simulink model "BloodPressure_ADC1"  (R2020b)
settings: Solver=ode15s  StartTime=0.0  StopTime=55  RelTol=1e-3  AbsTol=1e-3  EnableMultiTasking=on
libraries: fl_lib x33, nesl_utility x7, ee_lib x7
CloseFcn:
  | try,close(h1_elec_strain_gauge),end
  | clear h1_elec_strain_gauge
  | 
  | clear logsout_elec_strain_gauge
  | clear simlog_elec_strain_gauge
  | clear tout
Description:
  | Strain Gauge and Wheatstone Bridge
  | 
  | Copyright 2008-2018 The MathWorks, Inc.
settings Model: ExtModeAutoUpdateStatusClock=off  Creator=MathWorks  LastModifiedBy=bolic
settings SolverCC: AutoScaleAbsTol=off
settings DataIOCC: MaxDataPoints=10000  ReturnWorkspaceOutputs=off  SignalLoggingName=logsout_elec_strain_gauge  Refine=5
settings OptimizationCC: ExpressionDepthLimit=2147483647  InitFltsAndDblsToZero=on  LifeSpan=inf
settings DebuggingCC: SaveWithParameterizedLinksMsg=none  UnderspecifiedInitializationDetection=Classic  MergeDetectMultiDrivingBlocksExec=none  SignalResolutionControl=TryResolveAllWithWarning  FcnCallInpInsideContextMsg=warning  StateNameClashWarn=warning  SFUnexpectedBacktrackingDiag=warning  SFNoUnconditionalDefaultTransitionDiag=warning  SFExecutionAtInitializationDiag=none  ArithmeticOperatorsInVariantConditions=warning
settings HardwareCC: ProdBitPerPointer=32  ProdBitPerSizeT=32  ProdBitPerPtrDiffT=32  ProdLargestAtomicFloat=None  ProdIntDivRoundTo=Undefined  ProdEndianess=Unspecified  ProdWordSize=32  ProdHWDeviceType=32-bit Generic
settings ModelReferenceCC: PropagateSignalLabelsOutOfModel=off
settings SFSimCC: SimUseLocalCustomCode=off  CustomCodeUndefinedFunction=UseInterfaceOnly
settings RTWCC: RTWUseLocalCustomCode=off
settings CodeAppCC: StateflowObjectComments=on
settings GRTTargetCC: TargetFcnLib=ansi_tfl_tmw.mat  TargetLangStandard=C89/C90 (ANSI)  CombineOutputUpdateFcns=off  GRTInterface=on
settings ConfigComp: CovMetricSettings=dw  CovSaveCumulativeToWorkspaceVar=on  CovSaveSingleToWorkspaceVar=on  CovExternalEMLEnable=off  CovSFcnEnable=off
settings SimscapeCC: SimscapeLogType=all  SimscapeLogSimulationStatistics=on  SimscapeLogName=simlog_elec_strain_gauge  SimscapeLogDataHistory=10000

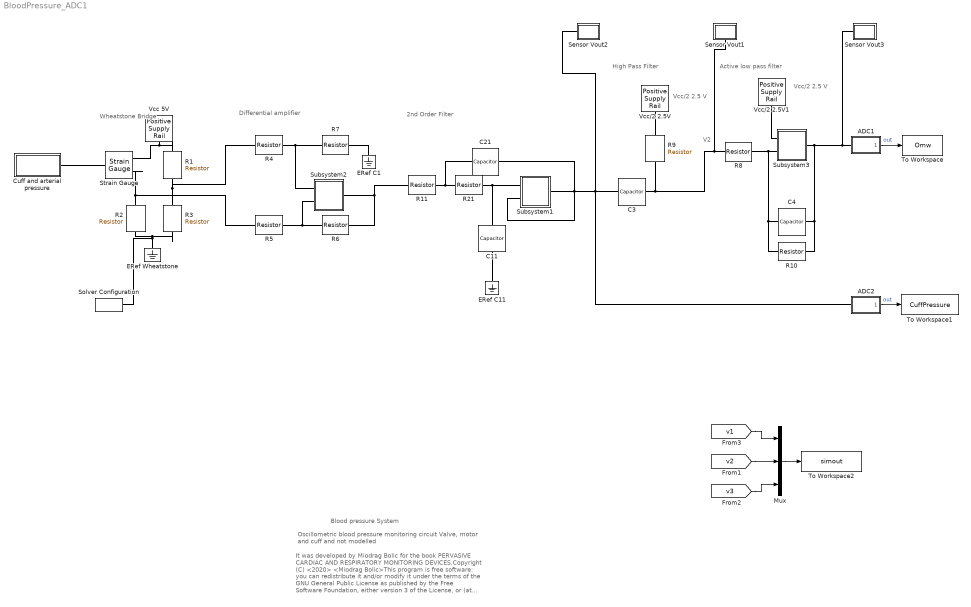
== system BloodPressure_ADC1 ==
  note: Vcc/2
      | 2.5 V
  note: It was developed by Miodrag Bolic for the book PERVASIVE CARDIAC AND RESPIRATORY MONITORING DEVICES.Copyright (C) <2020> <Miodrag Bolic>This program is free software: you can redistribute it and/or modify it under the terms of the GNU General Public License as published by the Free Software Foundation, either version 3 of the License, or (at your option) any later version. This program is distributed in the hope that it will be useful, but WITHOUT ANY WARRANTY; without even the implied warranty of MERCHANTABILITY or FITNESS FOR A PARTICULAR PURPOSE. See the GNU General Public License for more details <https://www.gnu.org/licenses/>.
  note: Wheatstone
      | Bridge
  note: Oscillometric blood pressure monitoring circuit
      | Valve, motor and cuff and not modelled
  note: 2nd Order Filter
  note: V2
  note: High Pass Filter
  note: Active low pass filter
  note: Blood pressure System
  note: Differential amplifier
  note: Vcc/2
      | 2.5 V
  ADC1 : Subsystem  mask(ADC){fs=200, N=12, vmax=5, ileak=1e-9, C=10e-12}
      mask prompts: fs "Sampling rate (Hz)"; N "Number of bits"; vmax "Input voltage for max output (V)"; ileak "Leakage current (A)"; C "Pin capacitance (F)"
      mask help: Simplified analog-to-digital converter
  ADC2 : Subsystem  mask(ADC){fs=200, N=12, vmax=5, ileak=1e-9, C=10e-12}
      mask prompts: fs "Sampling rate (Hz)"; N "Number of bits"; vmax "Input voltage for max output (V)"; ileak "Leakage current (A)"; C "Pin capacitance (F)"
      mask help: Simplified analog-to-digital converter
  C11 : fl_lib/Electrical/Electrical Elements/Capacitor  c=800 nF  r=0 Ohm  g=0 1/Ohm  i_specify=off  i_priority=High  i=0 A  i_nominal_specify=off  i_nominal_unit=A  i_nominal_value=1  v_specify=off  v_priority=High  v=0 V  v_nominal_specify=off  v_nominal_unit=V  v_nominal_value=1  vc_specify=off  vc_priority=High  vc=0 V  vc_nominal_specify=off  vc_nominal_unit=V  vc_nominal_value=1
      settings: AttributesFormatString=%<c> %<c_unit>  SourceProductName=Foundation Library
  C21 : fl_lib/Electrical/Electrical Elements/Capacitor  c=800 nF  r=0 Ohm  g=0 1/Ohm  i_specify=off  i_priority=High  i=0 A  i_nominal_specify=off  i_nominal_unit=A  i_nominal_value=1  v_specify=off  v_priority=High  v=0 V  v_nominal_specify=off  v_nominal_unit=V  v_nominal_value=1  vc_specify=off  vc_priority=High  vc=0 V  vc_nominal_specify=off  vc_nominal_unit=V  vc_nominal_value=1
      settings: AttributesFormatString=%<c>%<c_unit>  SourceProductName=Foundation Library
  C3 : fl_lib/Electrical/Electrical Elements/Capacitor  c=3.3 uF  r=1e-6 Ohm  g=0 1/Ohm  i_specify=off  i_priority=None  i=0 A  i_nominal_specify=off  i_nominal_unit=A  i_nominal_value=1  v_specify=off  v_priority=None  v=0 V  v_nominal_specify=off  v_nominal_unit=V  v_nominal_value=1  vc_specify=off  vc_priority=High  vc=0 V  vc_nominal_specify=off  vc_nominal_unit=V  vc_nominal_value=1
      settings: AttributesFormatString=%<c>%<c_unit>
  C4 : fl_lib/Electrical/Electrical Elements/Capacitor  c=0.6 nF  r=1e-6 Ohm  g=0 1/Ohm  i_specify=off  i_priority=None  i=0 A  i_nominal_specify=off  i_nominal_unit=A  i_nominal_value=1  v_specify=off  v_priority=None  v=0 V  v_nominal_specify=off  v_nominal_unit=V  v_nominal_value=1  vc_specify=off  vc_priority=High  vc=0 V  vc_nominal_specify=off  vc_nominal_unit=V  vc_nominal_value=1
      settings: AttributesFormatString=%<c>%<c_unit>
  Cuff and arterial pressure : Subsystem
  ERef C1 : fl_lib/Electrical/Electrical Elements/Electrical Reference
      settings: SourceProductName=Foundation Library
  ERef C11 : fl_lib/Electrical/Electrical Elements/Electrical Reference
      settings: SourceProductName=Foundation Library
  ERef Wheatstone : fl_lib/Electrical/Electrical Elements/Electrical Reference
      settings: SourceProductName=Foundation Library
  Mux : Mux  Inputs=3
  R1 : fl_lib/Electrical/Electrical Elements/Resistor  R=120 Ohm  i_specify=off  i_priority=High  i=0 A  i_nominal_specify=off  i_nominal_unit=A  i_nominal_value=1  v_specify=off  v_priority=High  v=0 V  v_nominal_specify=off  v_nominal_unit=V  v_nominal_value=1
      settings: AttributesFormatString=%<R> %<R_unit>  SourceProductName=Foundation Library
  R10 : fl_lib/Electrical/Electrical Elements/Resistor  R=15 MOhm  i_specify=off  i_priority=None  i=0 A  i_nominal_specify=off  i_nominal_unit=A  i_nominal_value=1  v_specify=off  v_priority=None  v=0 V  v_nominal_specify=off  v_nominal_unit=V  v_nominal_value=1
      settings: AttributesFormatString=%<R>%<R_unit>
  R11 : fl_lib/Electrical/Electrical Elements/Resistor  R=10 kOhm  i_specify=off  i_priority=High  i=0 A  i_nominal_specify=off  i_nominal_unit=A  i_nominal_value=1  v_specify=off  v_priority=High  v=0 V  v_nominal_specify=off  v_nominal_unit=V  v_nominal_value=1
      settings: AttributesFormatString=%<R> %<R_unit>  SourceProductName=Foundation Library
  R2 : fl_lib/Electrical/Electrical Elements/Resistor  R=120 Ohm  i_specify=off  i_priority=High  i=0 A  i_nominal_specify=off  i_nominal_unit=A  i_nominal_value=1  v_specify=off  v_priority=High  v=0 V  v_nominal_specify=off  v_nominal_unit=V  v_nominal_value=1
      settings: AttributesFormatString=%<R> %<R_unit>  SourceProductName=Foundation Library
  R21 : fl_lib/Electrical/Electrical Elements/Resistor  R="10  kOhm"  i_specify=off  i_priority=High  i=0 A  i_nominal_specify=off  i_nominal_unit=A  i_nominal_value=1  v_specify=off  v_priority=High  v=0 V  v_nominal_specify=off  v_nominal_unit=V  v_nominal_value=1
      settings: AttributesFormatString=%<R>%<R_unit>  SourceProductName=Foundation Library
  R3 : fl_lib/Electrical/Electrical Elements/Resistor  R=120 Ohm  i_specify=off  i_priority=High  i=0 A  i_nominal_specify=off  i_nominal_unit=A  i_nominal_value=1  v_specify=off  v_priority=High  v=0 V  v_nominal_specify=off  v_nominal_unit=V  v_nominal_value=1
      settings: AttributesFormatString=%<R> %<R_unit>  SourceProductName=Foundation Library
  R4 : fl_lib/Electrical/Electrical Elements/Resistor  R=100 Ohm  i_specify=off  i_priority=None  i=0 A  i_nominal_specify=off  i_nominal_unit=A  i_nominal_value=1  v_specify=off  v_priority=None  v=0 V  v_nominal_specify=off  v_nominal_unit=V  v_nominal_value=1
      settings: AttributesFormatString=%<R> %<R_unit>
  R5 : fl_lib/Electrical/Electrical Elements/Resistor  R=100 Ohm  i_specify=off  i_priority=None  i=0 A  i_nominal_specify=off  i_nominal_unit=A  i_nominal_value=1  v_specify=off  v_priority=None  v=0 V  v_nominal_specify=off  v_nominal_unit=V  v_nominal_value=1
      settings: AttributesFormatString=%<R> %<R_unit>
  R6 : fl_lib/Electrical/Electrical Elements/Resistor  R=10 kOhm  i_specify=off  i_priority=None  i=0 A  i_nominal_specify=off  i_nominal_unit=A  i_nominal_value=1  v_specify=off  v_priority=None  v=0 V  v_nominal_specify=off  v_nominal_unit=V  v_nominal_value=1
      settings: AttributesFormatString=%<R> %<R_unit>
  R7 : fl_lib/Electrical/Electrical Elements/Resistor  R=10 kOhm  i_specify=off  i_priority=None  i=0 A  i_nominal_specify=off  i_nominal_unit=A  i_nominal_value=1  v_specify=off  v_priority=None  v=0 V  v_nominal_specify=off  v_nominal_unit=V  v_nominal_value=1
      settings: AttributesFormatString=%<R> %<R_unit>
  R8 : fl_lib/Electrical/Electrical Elements/Resistor  R=250 kOhm  i_specify=off  i_priority=None  i=0 A  i_nominal_specify=off  i_nominal_unit=A  i_nominal_value=1  v_specify=off  v_priority=None  v=0 V  v_nominal_specify=off  v_nominal_unit=V  v_nominal_value=1
      settings: AttributesFormatString=%<R>%<R_unit>
  R9 : fl_lib/Electrical/Electrical Elements/Resistor  R=280 kOhm  i_specify=off  i_priority=None  i=0 A  i_nominal_specify=off  i_nominal_unit=A  i_nominal_value=1  v_specify=off  v_priority=None  v=0 V  v_nominal_specify=off  v_nominal_unit=V  v_nominal_value=1
      settings: AttributesFormatString=%<R>%<R_unit>
  Sensor Vout1 : Subsystem
      settings: PortSchema="{\"entries\":[{\"content\":{\"sides\":[{\"content\":{\"connectorIds\":[]},\"type\":\"ConnectorPlacement.EquallySpacedRectSide\",\"uuid\":\"78d8266e-4de3-447e-bfef-e5103e8c82e7\"},{\"content\":{\"connectorIds\":[],\"side\":\"RIGHT\"},\"type\":\"ConnectorPlacement.EquallySpacedRectSide\",\"uuid\":\"24c184c0-4d09-4cde-a27e-d86b719c7490\"},{\"content\":{\"connectorIds\":[],\"side\":\"TOP\"},\"type\":\"ConnectorPlacement.EquallySpacedRectSide\",\"uuid\":\"0a0b328c-c1d1-4c74-810b-0901e018f872\"},{\"content\":{\"connectorIds\":[\"RConn1\"],\"side\":\"BOTTOM\"},\"type\":\"ConnectorPlacement.EquallySpacedRectSide\",\"uuid\":\"04397490-2efd-4059-a127-c3271fe693a1\"},{\"content\":{\"connectorIds\":[],\"side\":\"HIDDEN\"},\"type\":\"ConnectorPlacement.EquallySpacedRectSide\",\"uuid\":\"df448a23-5d4a-4198-9543-ada33aea1d81\"}]},\"type\":\"ConnectorPlacement.EquallySpacedConnector\",\"uuid\":\"43700f0f-07d4-49b8-8a91-5fd2f7a62cdb\"}],\"packageUris\":[\"http://schema.mathworks.com/mf0/Connector/R2020b\"],\"version\":\"1.0\"}"
      mask Display: disp('V')
  Sensor Vout2 : Subsystem
      mask Display: disp('V')
  Sensor Vout3 : Subsystem
      mask Display: disp('V')
  Solver Configuration : nesl_utility/Solver Configuration  PhysicalDomain=network_engine_domain  SubClassName=solver  LeftPortType=input  RightPortType=generic  Tones=[]  Harmonics=[]  SimulateNoise=off  Profile=off  UseLocalSampling=off  EnableSwitchedLinearOptims=on  FrequencyDomain=off  UseCCode=off  RelTol=0.001  AbsTol=1e-06  MinStep=1e-09  ToWorkspace=off  RevertToSquareIcSolve=off  NumHomotopyIterations=100  PhasorMode=off  PhasorModeNumHarmonics=1  DoDC=off  ResidualTolerance=1e-9  UseLocalSolver=off  LocalSolverChoice=NE_BACKWARD_EULER_ADVANCER  LocalSolverSampleTime=.001  DoFixedCost=off  MaxNonlinIter=3  MaxModeIter=2  ComputeImpulses=off  ImpulseIterations=2  LinearAlgebra=auto  EquationFormulation=NE_TIME_EF  DelaysMemoryBudget=1024  AutomaticFiltering=on  FilteringTimeConstant=0.001  PartitionStorageMethod=AS_NEEDED  PartitionMemoryBudget=1024  PartitionMethod=FAST
  Strain Gauge : ee_lib/Sensors & Transducers/Strain Gauge  R=120 Ohm  K=2
      settings: SourceProductBaseCode=PS  InternalSimscapePortConfiguration="{\"Bottom\":[],\"Left\":[{\"id\":\"E\",\"label\":\"E\",\"type\":\"input\"}],\"Right\":[{\"id\":\"p\",\"label\":\"+\",\"type\":\"foundation.electrical.electrical\"},{\"id\":\"n\",\"label\":\"-\",\"type\":\"foundation.electrical.electrical\"}],\"Top\":[]}"
  Subsystem1 : Subsystem
      mask Display: image('op_amp_plus_up.png')
  Subsystem2 : Subsystem
      mask Display: image('op_amp_plus_up.png')
  Subsystem3 : Subsystem
      mask Display: image('op_amp_plus_up.png')
  To Workspace : ToWorkspace  VariableName=Omw  SaveFormat=Timeseries  SampleTime=0.001
  To Workspace1 : ToWorkspace  VariableName=CuffPressure  SaveFormat=Timeseries  SampleTime=0.001
  To Workspace2 : ToWorkspace  VariableName=simout  SaveFormat=Timeseries  SampleTime=-1
  Vcc 5V : ee_lib/Sources/Positive Supply Rail  v0=5 V
      settings: SourceProductBaseCode=PS  InternalSimscapePortConfiguration="{\"Bottom\":[],\"Left\":[],\"Right\":[{\"id\":\"p\",\"label\":\"\",\"type\":\"foundation.electrical.electrical\"}],\"Top\":[]}"
  Vcc/2 2.5V : ee_lib/Sources/Positive Supply Rail  v0=2.5 V
      settings: SourceProductBaseCode=PS  InternalSimscapePortConfiguration="{\"Bottom\":[],\"Left\":[],\"Right\":[{\"id\":\"p\",\"label\":\"\",\"type\":\"foundation.electrical.electrical\"}],\"Top\":[]}"
  Vcc/2 2.5V1 : ee_lib/Sources/Positive Supply Rail  v0=2.5 V
      settings: SourceProductBaseCode=PS  InternalSimscapePortConfiguration="{\"Bottom\":[],\"Left\":[],\"Right\":[{\"id\":\"p\",\"label\":\"\",\"type\":\"foundation.electrical.electrical\"}],\"Top\":[]}"
  wires:
  ADC1/1(Out_Int) -> To Workspace/1  "out"
  ADC2/1(Out_Int) -> To Workspace1/1  "out"
  Mux/1 -> To Workspace2/1
  [v1] -> Mux/1
  [v2] -> Mux/2
  [v3] -> Mux/3
  connections:
  R1/LConn1 -- Strain Gauge/RConn1 -- Vcc 5V/RConn1
  R3/RConn1 -- R2/RConn1 -- Solver Configuration/RConn1 -- ERef Wheatstone/LConn1
  R21/RConn1 -- Subsystem1/LConn1 -- C11/LConn1
  R21/LConn1 -- R11/RConn1 -- C21/LConn1
  C21/RConn1 -- Subsystem1/LConn2 -- Subsystem1/RConn1 -- Sensor Vout2/LConn1 -- C3/LConn1 -- ADC2/LConn1
  R10/RConn1 -- Subsystem3/RConn1 -- Sensor Vout3/LConn1 -- ADC1/LConn1 -- C4/LConn1
  C3/RConn1 -- R9/RConn1 -- Sensor Vout1/RConn1 -- R8/LConn1
  R8/RConn1 -- Subsystem3/LConn2 -- R10/LConn1 -- C4/RConn1
  Vcc/2 2.5V1/RConn1 -- Subsystem3/LConn1
  Vcc/2 2.5V/RConn1 -- R9/LConn1
  Cuff and arterial pressure/RConn1 -- Strain Gauge/LConn1
  ERef C1/LConn1 -- R7/RConn1
  R5/RConn1 -- Subsystem2/LConn2 -- R6/LConn1
  R11/LConn1 -- Subsystem2/RConn1 -- R6/RConn1
  R1/RConn1 -- R4/LConn1 -- R3/LConn1
  R4/RConn1 -- Subsystem2/LConn1 -- R7/LConn1
  Strain Gauge/RConn2 -- R5/LConn1 -- R2/LConn1
  ERef C11/LConn1 -- C11/RConn1

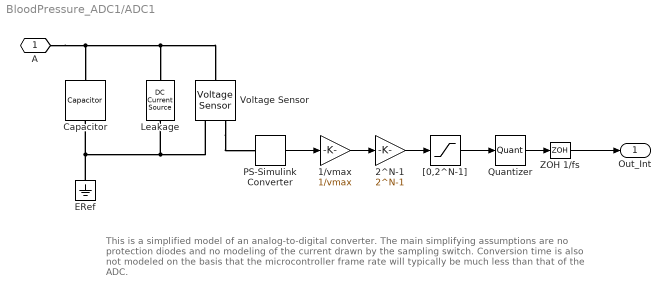
== system BloodPressure_ADC1/ADC1 ==
  note: This is a simplified model of an analog-to-digital converter. The main simplifying assumptions
      | are no protection diodes and no modeling of the current drawn by the sampling switch.
      | Conversion time is also not modeled on the basis that the microcontroller frame rate will
      | typically be much less than that of the ADC.
  1/vmax : Gain  Gain=1/vmax
  2^N-1 : Gain  Gain=2^N-1
  Capacitor : fl_lib/Electrical/Electrical Elements/Capacitor  c=1e-6 F  r=1e-6 Ohm  g=0 1/Ohm  i_specify=off  i_priority=High  i=0 A  i_nominal_specify=off  i_nominal_unit=A  i_nominal_value=1  v_specify=off  v_priority=High  v=0 V  v_nominal_specify=off  v_nominal_unit=V  v_nominal_value=1  vc_specify=on  vc_priority=High  vc=0 V  vc_nominal_specify=off  vc_nominal_unit=V  vc_nominal_value=1
      settings: SourceProductName=Foundation Library
  ERef : fl_lib/Electrical/Electrical Elements/Electrical Reference
      settings: SourceProductName=Foundation Library
  Leakage : fl_lib/Electrical/Electrical Sources/DC Current Source  i0=ileak A
      settings: SourceProductName=Foundation Library  InternalSimscapePortConfiguration="{\"Bottom\":[],\"Left\":[{\"id\":\"p\",\"label\":\"\",\"type\":\"foundation.electrical.electrical\"}],\"Right\":[{\"id\":\"n\",\"label\":\"\",\"type\":\"foundation.electrical.electrical\"}],\"Top\":[]}"
  PS-Simulink Converter : nesl_utility/PS-Simulink Converter  PhysicalDomain=network_engine_domain  SubClassName=ps_output  LeftPortType=input  RightPortType=output  PseudoPeriodic=off  Frequencies=[]  Unit=V  AffineConversion=off
  Quantizer : Quantizer  QuantizationInterval=1
  Voltage Sensor : fl_lib/Electrical/Electrical Sensors/Voltage Sensor
      settings: SourceProductName=Foundation Library
  ZOH 1/fs : ZeroOrderHold  SampleTime=1/fs
  "[0,2^N-1]" : Saturate  UpperLimit=2^N-1  LowerLimit=0
  A : PMIOPort  Side=Left
  Out_Int : Outport  VectorParamsAs1DForOutWhenUnconnected=off
  wires:
  "[0,2^N-1]"/1 -> Quantizer/1
  1/vmax/1 -> 2^N-1/1
  2^N-1/1 -> "[0,2^N-1]"/1
  PS-Simulink Converter/1 -> 1/vmax/1
  ZOH 1/fs/1 -> Out_Int/1
  Quantizer/1 -> ZOH 1/fs/1
  connections:
  A/RConn1 -- Voltage Sensor/LConn1 -- Leakage/RConn1 -- Capacitor/LConn1
  ERef/LConn1 -- Voltage Sensor/RConn2 -- Leakage/LConn1 -- Capacitor/RConn1
  Voltage Sensor/RConn1 -- PS-Simulink Converter/LConn1

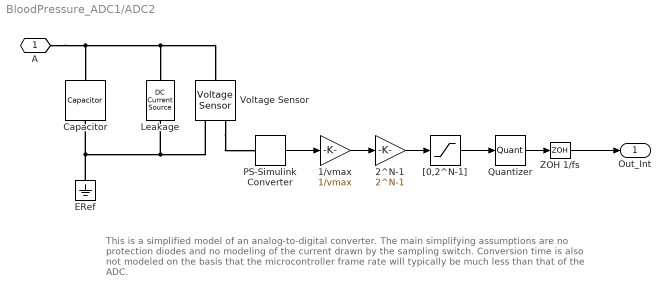
== system BloodPressure_ADC1/ADC2 ==
  note: This is a simplified model of an analog-to-digital converter. The main simplifying assumptions
      | are no protection diodes and no modeling of the current drawn by the sampling switch.
      | Conversion time is also not modeled on the basis that the microcontroller frame rate will
      | typically be much less than that of the ADC.
  1/vmax : Gain  Gain=1/vmax
  2^N-1 : Gain  Gain=2^N-1
  Capacitor : fl_lib/Electrical/Electrical Elements/Capacitor  c=1e-6 F  r=1e-6 Ohm  g=0 1/Ohm  i_specify=off  i_priority=High  i=0 A  i_nominal_specify=off  i_nominal_unit=A  i_nominal_value=1  v_specify=off  v_priority=High  v=0 V  v_nominal_specify=off  v_nominal_unit=V  v_nominal_value=1  vc_specify=on  vc_priority=High  vc=0 V  vc_nominal_specify=off  vc_nominal_unit=V  vc_nominal_value=1
      settings: SourceProductName=Foundation Library
  ERef : fl_lib/Electrical/Electrical Elements/Electrical Reference
      settings: SourceProductName=Foundation Library
  Leakage : fl_lib/Electrical/Electrical Sources/DC Current Source  i0=ileak A
      settings: SourceProductName=Foundation Library  InternalSimscapePortConfiguration="{\"Bottom\":[],\"Left\":[{\"id\":\"p\",\"label\":\"\",\"type\":\"foundation.electrical.electrical\"}],\"Right\":[{\"id\":\"n\",\"label\":\"\",\"type\":\"foundation.electrical.electrical\"}],\"Top\":[]}"
  PS-Simulink Converter : nesl_utility/PS-Simulink Converter  PhysicalDomain=network_engine_domain  SubClassName=ps_output  LeftPortType=input  RightPortType=output  PseudoPeriodic=off  Frequencies=[]  Unit=V  AffineConversion=off
  Quantizer : Quantizer  QuantizationInterval=1
  Voltage Sensor : fl_lib/Electrical/Electrical Sensors/Voltage Sensor
      settings: SourceProductName=Foundation Library
  ZOH 1/fs : ZeroOrderHold  SampleTime=1/fs
  "[0,2^N-1]" : Saturate  UpperLimit=2^N-1  LowerLimit=0
  A : PMIOPort  Side=Left
  Out_Int : Outport  VectorParamsAs1DForOutWhenUnconnected=off
  wires:
  "[0,2^N-1]"/1 -> Quantizer/1
  1/vmax/1 -> 2^N-1/1
  2^N-1/1 -> "[0,2^N-1]"/1
  PS-Simulink Converter/1 -> 1/vmax/1
  ZOH 1/fs/1 -> Out_Int/1
  Quantizer/1 -> ZOH 1/fs/1
  connections:
  A/RConn1 -- Voltage Sensor/LConn1 -- Leakage/RConn1 -- Capacitor/LConn1
  ERef/LConn1 -- Voltage Sensor/RConn2 -- Leakage/LConn1 -- Capacitor/RConn1
  Voltage Sensor/RConn1 -- PS-Simulink Converter/LConn1

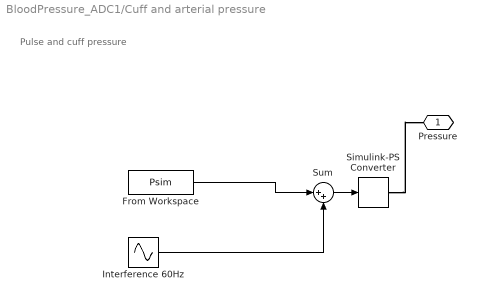
== system BloodPressure_ADC1/Cuff and arterial pressure ==
  note: Pulse and cuff pressure
  From Workspace : FromWorkspace  VariableName=Psim  SampleTime=0.005
  Interference 60Hz : Sin  Amplitude=0.00001  Frequency=120*pi  SampleTime=0.001
  Simulink-PS Converter : nesl_utility/Simulink-PS Converter  PhysicalDomain=network_engine_domain  SubClassName=ps_input  LeftPortType=input  RightPortType=output  PseudoPeriodic=off  Frequencies=[]  NoiseDistribution=none  NoiseParameters=[]  Unit=1  AffineConversion=off  FilteringAndDerivatives=zero  SimscapeFilterOrder=1  InputFilterTimeConstant=.001  UdotUserProvided=0
  Sum : Sum  Inputs=|++
  Pressure : PMIOPort  Side=Right
  wires:
  Interference 60Hz/1 -> Sum/2
  From Workspace/1 -> Sum/1
  Sum/1 -> Simulink-PS Converter/1
  connections:
  Simulink-PS Converter/RConn1 -- Pressure/RConn1

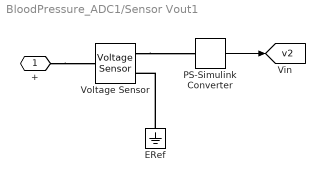
== system BloodPressure_ADC1/Sensor Vout1 ==
  ERef : fl_lib/Electrical/Electrical Elements/Electrical Reference
      settings: SourceProductName=Foundation Library
  PS-Simulink Converter : nesl_utility/PS-Simulink Converter  PhysicalDomain=network_engine_domain  SubClassName=ps_output  LeftPortType=input  RightPortType=output  PseudoPeriodic=off  Frequencies=[]  Unit=1  AffineConversion=off
      settings: SourceProductName=Utilities
  Voltage Sensor : fl_lib/Electrical/Electrical Sensors/Voltage Sensor
      settings: SourceProductName=Foundation Library
  + : PMIOPort  Side=Right
  tag scope: v2=global
  wires:
  PS-Simulink Converter/1 -> [v2]
  connections:
  ERef/LConn1 -- Voltage Sensor/RConn2
  Voltage Sensor/RConn1 -- PS-Simulink Converter/LConn1
  +/RConn1 -- Voltage Sensor/LConn1

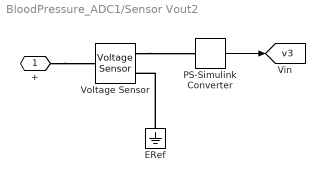
== system BloodPressure_ADC1/Sensor Vout2 ==
  ERef : fl_lib/Electrical/Electrical Elements/Electrical Reference
      settings: SourceProductName=Foundation Library
  PS-Simulink Converter : nesl_utility/PS-Simulink Converter  PhysicalDomain=network_engine_domain  SubClassName=ps_output  LeftPortType=input  RightPortType=output  PseudoPeriodic=off  Frequencies=[]  Unit=1  AffineConversion=off
      settings: SourceProductName=Utilities
  Voltage Sensor : fl_lib/Electrical/Electrical Sensors/Voltage Sensor
      settings: SourceProductName=Foundation Library
  + : PMIOPort  Side=Left
  tag scope: v3=global
  wires:
  PS-Simulink Converter/1 -> [v3]
  connections:
  ERef/LConn1 -- Voltage Sensor/RConn2
  Voltage Sensor/RConn1 -- PS-Simulink Converter/LConn1
  +/RConn1 -- Voltage Sensor/LConn1

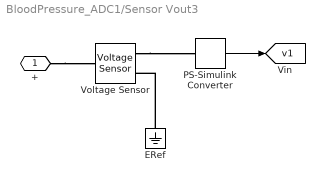
== system BloodPressure_ADC1/Sensor Vout3 ==
  ERef : fl_lib/Electrical/Electrical Elements/Electrical Reference
      settings: SourceProductName=Foundation Library
  PS-Simulink Converter : nesl_utility/PS-Simulink Converter  PhysicalDomain=network_engine_domain  SubClassName=ps_output  LeftPortType=input  RightPortType=output  PseudoPeriodic=off  Frequencies=[]  Unit=1  AffineConversion=off
      settings: SourceProductName=Utilities
  Voltage Sensor : fl_lib/Electrical/Electrical Sensors/Voltage Sensor
      settings: SourceProductName=Foundation Library
  + : PMIOPort  Side=Left
  tag scope: v1=global
  wires:
  PS-Simulink Converter/1 -> [v1]
  connections:
  ERef/LConn1 -- Voltage Sensor/RConn2
  Voltage Sensor/RConn1 -- PS-Simulink Converter/LConn1
  +/RConn1 -- Voltage Sensor/LConn1

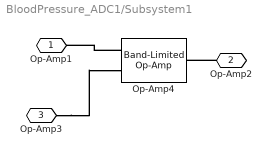
== system BloodPressure_ADC1/Subsystem1 ==
  Op-Amp4 : ee_lib/Integrated Circuits/Band-Limited Op-Amp  A=50000  Rin=6e+6 Ohm  Rout=100 Ohm  Vmin=0 V  Vmax=5 V  Vdotmax=0.7e6 V/s  f=1.5e+6 Hz  V0=0 V
      settings: SourceProductBaseCode=PS
  Op-Amp1 : PMIOPort  Side=Left
  Op-Amp2 : PMIOPort  Port=2  Side=Right
  Op-Amp3 : PMIOPort  Port=3  Side=Left
  connections:
  Op-Amp4/LConn1 -- Op-Amp1/RConn1
  Op-Amp3/RConn1 -- Op-Amp4/LConn2
  Op-Amp2/RConn1 -- Op-Amp4/RConn1

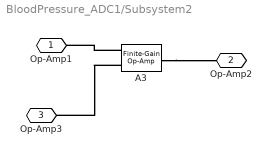
== system BloodPressure_ADC1/Subsystem2 ==
  A3 : ee_lib/Integrated Circuits/Finite-Gain Op-Amp  A=1000  Rin=1e+6 Ohm  Rout=100 Ohm  Vmin=-5 V  Vmax=5 V  noise_mode=0  v_noise=30e-9 V/Hz^0.50000  noise_prm=1  i_noise=0.5e-12 A/Hz^0.50000  ip_noise=0.5e-12 A/Hz^0.50000  in_noise=0.5e-12 A/Hz^0.50000  sample_time=1e-3 s  repeatability=1  auto_seed_v=2264060836  auto_seed_ip=1964622691  auto_seed_in=3759692387  user_seed_v=0  user_seed_ip=0  user_seed_in=0
      settings: SourceProductBaseCode=PS  InternalSimscapePortConfiguration="{\"Bottom\":[],\"Left\":[{\"id\":\"p\",\"label\":\"+\",\"type\":\"foundation.electrical.electrical\"},{\"id\":\"n\",\"label\":\"-\",\"type\":\"foundation.electrical.electrical\"}],\"Right\":[{\"id\":\"out\",\"label\":\"\",\"type\":\"foundation.electrical.electrical\"}],\"Top\":[]}"
  Op-Amp1 : PMIOPort  Side=Left
  Op-Amp2 : PMIOPort  Port=2  Side=Right
  Op-Amp3 : PMIOPort  Port=3  Side=Left
  connections:
  A3/LConn1 -- Op-Amp1/RConn1
  A3/LConn2 -- Op-Amp3/RConn1
  A3/RConn1 -- Op-Amp2/RConn1

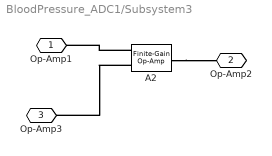
== system BloodPressure_ADC1/Subsystem3 ==
  A2 : ee_lib/Integrated Circuits/Finite-Gain Op-Amp  A=4.7e6  Rin=1e+6 Ohm  Rout=100 Ohm  Vmin=0 V  Vmax=5 V  noise_mode=0  v_noise=30e-9 V/Hz^0.50000  noise_prm=1  i_noise=0.5e-12 A/Hz^0.50000  ip_noise=0.5e-12 A/Hz^0.50000  in_noise=0.5e-12 A/Hz^0.50000  sample_time=1e-3 s  repeatability=1  auto_seed_v=1241522882  auto_seed_ip=2885394099  auto_seed_in=2985605712  user_seed_v=0  user_seed_ip=0  user_seed_in=0
      settings: SourceProductBaseCode=PS  InternalSimscapePortConfiguration="{\"Bottom\":[],\"Left\":[{\"id\":\"p\",\"label\":\"+\",\"type\":\"foundation.electrical.electrical\"},{\"id\":\"n\",\"label\":\"-\",\"type\":\"foundation.electrical.electrical\"}],\"Right\":[{\"id\":\"out\",\"label\":\"\",\"type\":\"foundation.electrical.electrical\"}],\"Top\":[]}"
  Op-Amp1 : PMIOPort  Side=Left
  Op-Amp2 : PMIOPort  Port=2  Side=Right
  Op-Amp3 : PMIOPort  Port=3  Side=Left
  connections:
  A2/LConn1 -- Op-Amp1/RConn1
  A2/LConn2 -- Op-Amp3/RConn1
  A2/RConn1 -- Op-Amp2/RConn1
